simulink model "matcher_simu_old"  (R2019b)
settings: Solver=FixedStepDiscrete  StartTime=0.0  StopTime=N_sym  RelTol=1e-3
InitFcn:
  | %% DSPBuilder Start
  | alt_dspbuilder_update_model(bdroot)
  | %% DSPBuilder End
  | 
  | matcher_init
StartFcn:
  | %% DSPBuilder Start
  | alt_dspbuilder_hdlimport_prepare_for_simulation(bdroot)
  | %% DSPBuilder End
StopFcn:
  | matcher_analysis
libraries: allblocks_alteradspbuilder2 x13, dspsrcs4 x2
settings Model: Creator=vboxuser  LastModifiedBy=vboxuser
settings DataIOCC: SaveFormat=Array

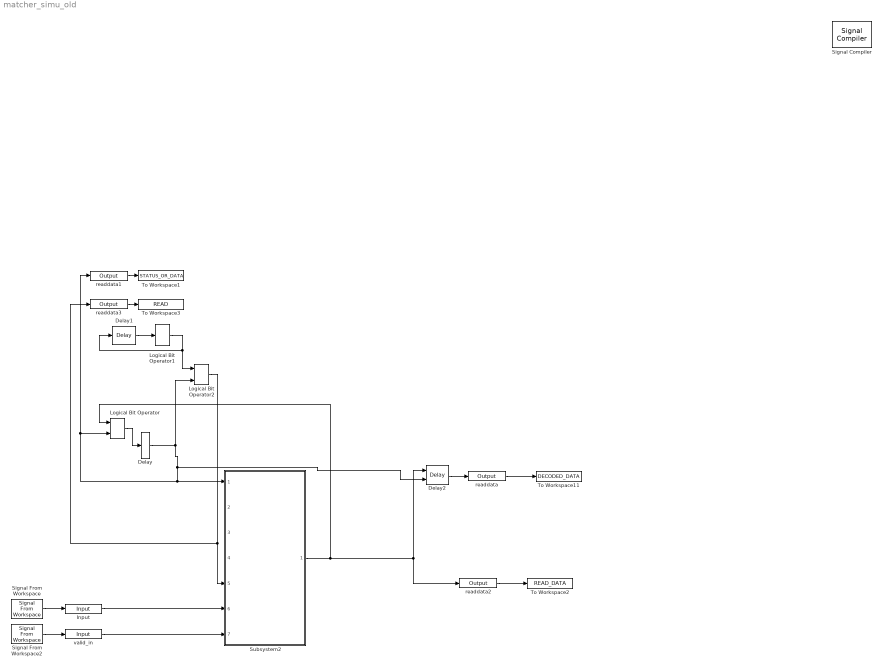
== system matcher_simu_old ==
  Delay : allblocks_alteradspbuilder2/Delay  pipeline=1  pipeline_display=1  ClockPhase=1  use_ena=off  use_sclr=off  allowFloatingPointOverride=on  logOutputs=off  logFile=C:\Users\vboxuser\Documents\MATLAB\serializer\system2\tb_matcher_simu_old\matcher%5Fsimu%5Fold_Delay.fixedpointlog  use_init=off  reset_value=1
  Delay1 : allblocks_alteradspbuilder2/Delay  pipeline=1  pipeline_display=1  ClockPhase=1  use_ena=off  use_sclr=off  allowFloatingPointOverride=on  logOutputs=off  logFile=C:\Users\vboxuser\Documents\MATLAB\serializer\system2\tb_matcher_simu_old\matcher%5Fsimu%5Fold_Delay1.fixedpointlog  use_init=off  reset_value=1
  Delay2 : allblocks_alteradspbuilder2/Delay  pipeline=1  pipeline_display=1  ClockPhase=1  use_ena=on  use_sclr=off  allowFloatingPointOverride=on  logOutputs=off  logFile=C:\Users\vboxuser\Documents\MATLAB\serializer\system2\tb_matcher_simu_old\matcher%5Fsimu%5Fold_Delay2.fixedpointlog  use_init=off  reset_value=1
  Input : allblocks_alteradspbuilder2/Input  iofile=C:\Users\vboxuser\Documents\MATLAB\serializer\system2\tb_matcher_simu_old\matcher%5Fsimu%5Fold_Input.salt  BusType=Single Bit  bwl=8  bwr=0  SpecifyClock=off  PORTTYPE=Input  externalType=Inferred  allowFloatingPointOverride=on  logOutputs=off
  Logical Bit Operator : allblocks_alteradspbuilder2/Logical Bit Operator  LogicalOperator=OR  user_inputs=2  pipeline_display=0
  Logical Bit Operator1 : allblocks_alteradspbuilder2/Logical Bit Operator  LogicalOperator=NOT  user_inputs=2  pipeline_display=0
  Logical Bit Operator2 : allblocks_alteradspbuilder2/Logical Bit Operator  LogicalOperator=AND  user_inputs=2  pipeline_display=0
  Signal Compiler : allblocks_alteradspbuilder2/Signal Compiler  DeviceFamily=Cyclone IV E  DeviceName=AUTO  DisableEarlyHDLGeneration=off  EnableSignalTap=off  SignalTapDepth=128  UseBoardBlock=off  StpUseDefaultClock=on  StpClock=Clock  ExportDir=D:\pliki-programow\intel\18.1\quartus\dsp_builder  MAX10_ProgrammingMode=Internal Flash (SDM) Single Boot
  Signal From Workspace : dspsrcs4/Signal From Workspace  X=data_in  Ts=1  nsamps=1  OutputAfterFinalValue=Setting to zero  ignoreOrWarnInputAndFrameLengths=off  OutputFrames=off
  Signal From Workspace2 : dspsrcs4/Signal From Workspace  X=valid_in  Ts=1  nsamps=1  OutputAfterFinalValue=Setting to zero  ignoreOrWarnInputAndFrameLengths=off  OutputFrames=off
  Subsystem2 : Subsystem  ReferencedSubsystem=AP5
  To Workspace1 : ToWorkspace  VariableName=STATUS_OR_DATA  SampleTime=-1
      settings: Save2DSignal=2-D array (concatenate along first dimension)
  To Workspace11 : ToWorkspace  VariableName=DECODED_DATA  SampleTime=-1
      settings: Save2DSignal=2-D array (concatenate along first dimension)
  To Workspace2 : ToWorkspace  VariableName=READ_DATA  SampleTime=-1
      settings: Save2DSignal=2-D array (concatenate along first dimension)
  To Workspace3 : ToWorkspace  VariableName=READ  SampleTime=-1
      settings: Save2DSignal=2-D array (concatenate along first dimension)
  readdata : allblocks_alteradspbuilder2/Output  iofile=C:\Users\vboxuser\Documents\MATLAB\serializer\system2\tb_matcher_simu_old\matcher%5Fsimu%5Fold_readdata.capture  BusType=Unsigned Integer  bwl=32  bwr=0  externalType=Inferred  PORTTYPE=Output  allowFloatingPointOverride=on  logOutputs=off
  readdata1 : allblocks_alteradspbuilder2/Output  iofile=C:\Users\vboxuser\Documents\MATLAB\serializer\system2\tb_matcher_simu_old\matcher%5Fsimu%5Fold_readdata1.capture  BusType=Single Bit  bwl=32  bwr=0  externalType=Inferred  PORTTYPE=Output  allowFloatingPointOverride=on  logOutputs=off
  readdata2 : allblocks_alteradspbuilder2/Output  iofile=C:\Users\vboxuser\Documents\MATLAB\serializer\system2\tb_matcher_simu_old\matcher%5Fsimu%5Fold_readdata2.capture  BusType=Unsigned Integer  bwl=32  bwr=0  externalType=Inferred  PORTTYPE=Output  allowFloatingPointOverride=on  logOutputs=off
  readdata3 : allblocks_alteradspbuilder2/Output  iofile=C:\Users\vboxuser\Documents\MATLAB\serializer\system2\tb_matcher_simu_old\matcher%5Fsimu%5Fold_readdata3.capture  BusType=Single Bit  bwl=32  bwr=0  externalType=Inferred  PORTTYPE=Output  allowFloatingPointOverride=on  logOutputs=off
  valid_in : allblocks_alteradspbuilder2/Input  iofile=C:\Users\vboxuser\Documents\MATLAB\serializer\system2\tb_matcher_simu_old\matcher%5Fsimu%5Fold_valid%5Fin.salt  BusType=Single Bit  bwl=8  bwr=0  SpecifyClock=off  PORTTYPE=Input  externalType=Inferred  allowFloatingPointOverride=on  logOutputs=off
  wires:
  Signal From Workspace/1 -> Input/1
  Signal From Workspace2/1 -> valid_in/1
  Input/1 -> Subsystem2/6
  valid_in/1 -> Subsystem2/7
  Subsystem2/1 -> readdata2/1, Delay2/1, Logical Bit Operator/1
  Logical Bit Operator/1 -> Delay/1
  Delay1/1 -> Logical Bit Operator1/1
  Logical Bit Operator1/1 -> Logical Bit Operator2/1, Delay1/1
  Delay/1 -> Delay2/2, Subsystem2/1, readdata1/1, Logical Bit Operator/2, Logical Bit Operator2/2
  Delay2/1 -> readdata/1
  readdata/1 -> To Workspace11/1
  readdata1/1 -> To Workspace1/1
  readdata2/1 -> To Workspace2/1
  readdata3/1 -> To Workspace3/1
  Logical Bit Operator2/1 -> Subsystem2/5, readdata3/1
